simulink model "Filter_PQ_Data"  (R2018a)
settings: Solver=ode45  StartTime=0.0  StopTime=5  RelTol=1e-3  EnableMultiTasking=on
Description:
  | Copyright 2014-2018 The MathWorks, Inc.
settings Model: Creator=smiller  LastModifiedBy=smiller
settings DataIOCC: LimitDataPoints=on  SaveFormat=Array
settings OptimizationCC: LifeSpan=inf
settings DebuggingCC: UnderspecifiedInitializationDetection=Classic  MergeDetectMultiDrivingBlocksExec=none  SolverPrmCheckMsg=warning  AllowSymbolicDim=off  StateNameClashWarn=warning  SFUnexpectedBacktrackingDiag=warning  SFNoUnconditionalDefaultTransitionDiag=warning  SFExecutionAtInitializationDiag=none
settings HardwareCC: ProdBitPerPointer=32  ProdBitPerSizeT=32  ProdBitPerPtrDiffT=32  ProdLargestAtomicFloat=None  ProdIntDivRoundTo=Undefined  ProdEndianess=Unspecified  ProdWordSize=32  ProdHWDeviceType=32-bit Generic
settings ModelReferenceCC: PropagateSignalLabelsOutOfModel=off
settings CodeAppCC: StateflowObjectComments=on
settings GRTTargetCC: TargetLangStandard=C89/C90 (ANSI)  GeneratePreprocessorConditionals=Disable all
settings ConfigComp: CovMetricSettings=dw  CovHtmlReporting=on  CovSaveCumulativeToWorkspaceVar=on  CovSaveSingleToWorkspaceVar=on  CovExternalEMLEnable=off  CovSFcnEnable=off

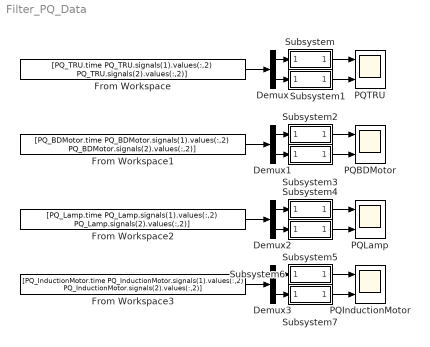
== system Filter_PQ_Data ==
  Demux{,1..3} (4 alike) : Demux  Outputs=2
  From Workspace : FromWorkspace  VariableName=[PQ_TRU.time PQ_TRU.signals(1).values(:,2) PQ_TRU.signals(2).values(:,2)]  SampleTime=0
  From Workspace1 : FromWorkspace  VariableName=[PQ_BDMotor.time PQ_BDMotor.signals(1).values(:,2) PQ_BDMotor.signals(2).values(:,2)]  SampleTime=0
  From Workspace2 : FromWorkspace  VariableName=[PQ_Lamp.time PQ_Lamp.signals(1).values(:,2) PQ_Lamp.signals(2).values(:,2)]  SampleTime=0
  From Workspace3 : FromWorkspace  VariableName=[PQ_InductionMotor.time PQ_InductionMotor.signals(1).values(:,2) PQ_InductionMotor.signals(2).values(:,2)]  SampleTime=0
  PQBDMotor : Scope  NumInputPorts=2
  PQInductionMotor : Scope  NumInputPorts=2
  PQLamp : Scope  NumInputPorts=2
  PQTRU : Scope  NumInputPorts=2
  Subsystem : Subsystem
  Subsystem1 : Subsystem
  Subsystem2 : Subsystem
  Subsystem3 : Subsystem
  Subsystem4 : Subsystem
  Subsystem5 : Subsystem
  Subsystem6 : Subsystem
  Subsystem7 : Subsystem
  wires:
  Subsystem/1(Out1) -> PQTRU/1
  Subsystem1/1(Out1) -> PQTRU/2
  Subsystem2/1(Out1) -> PQBDMotor/1
  Subsystem3/1(Out1) -> PQBDMotor/2
  From Workspace/1 -> Demux/1
  Demux/1 -> Subsystem/1(In1)
  Demux/2 -> Subsystem1/1(In1)
  From Workspace1/1 -> Demux1/1
  Demux1/1 -> Subsystem2/1(In1)
  Demux1/2 -> Subsystem3/1(In1)
  Subsystem4/1(Out1) -> PQLamp/1
  Subsystem5/1(Out1) -> PQLamp/2
  From Workspace2/1 -> Demux2/1
  Demux2/1 -> Subsystem4/1(In1)
  Demux2/2 -> Subsystem5/1(In1)
  Subsystem6/1(Out1) -> PQInductionMotor/1
  Subsystem7/1(Out1) -> PQInductionMotor/2
  From Workspace3/1 -> Demux3/1
  Demux3/1 -> Subsystem6/1(In1)
  Demux3/2 -> Subsystem7/1(In1)

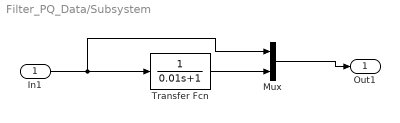
== system Filter_PQ_Data/Subsystem ==
  In1 : Inport
  Mux : Mux  Inputs=2
  Transfer Fcn : TransferFcn  Denominator=[0.01 1]
  Out1 : Outport
  wires:
  Mux/1 -> Out1/1
  In1/1 -> Mux/1, Transfer Fcn/1
  Transfer Fcn/1 -> Mux/2

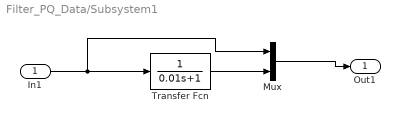
== system Filter_PQ_Data/Subsystem1 ==
  In1 : Inport
  Mux : Mux  Inputs=2
  Transfer Fcn : TransferFcn  Denominator=[0.01 1]
  Out1 : Outport
  wires:
  Transfer Fcn/1 -> Mux/2
  In1/1 -> Transfer Fcn/1, Mux/1
  Mux/1 -> Out1/1

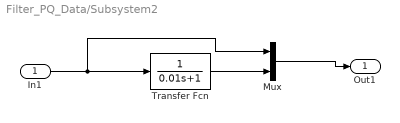
== system Filter_PQ_Data/Subsystem2 ==
  In1 : Inport
  Mux : Mux  Inputs=2
  Transfer Fcn : TransferFcn  Denominator=[0.01 1]
  Out1 : Outport
  wires:
  Transfer Fcn/1 -> Mux/2
  In1/1 -> Transfer Fcn/1, Mux/1
  Mux/1 -> Out1/1

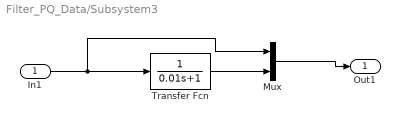
== system Filter_PQ_Data/Subsystem3 ==
  In1 : Inport
  Mux : Mux  Inputs=2
  Transfer Fcn : TransferFcn  Denominator=[0.01 1]
  Out1 : Outport
  wires:
  Mux/1 -> Out1/1
  In1/1 -> Mux/1, Transfer Fcn/1
  Transfer Fcn/1 -> Mux/2

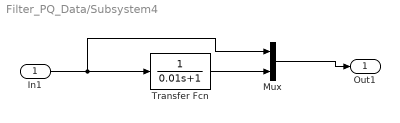
== system Filter_PQ_Data/Subsystem4 ==
  In1 : Inport
  Mux : Mux  Inputs=2
  Transfer Fcn : TransferFcn  Denominator=[0.01 1]
  Out1 : Outport
  wires:
  Mux/1 -> Out1/1
  In1/1 -> Mux/1, Transfer Fcn/1
  Transfer Fcn/1 -> Mux/2

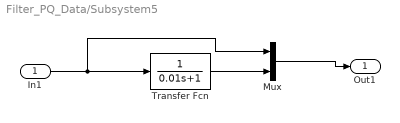
== system Filter_PQ_Data/Subsystem5 ==
  In1 : Inport
  Mux : Mux  Inputs=2
  Transfer Fcn : TransferFcn  Denominator=[0.01 1]
  Out1 : Outport
  wires:
  Transfer Fcn/1 -> Mux/2
  In1/1 -> Transfer Fcn/1, Mux/1
  Mux/1 -> Out1/1

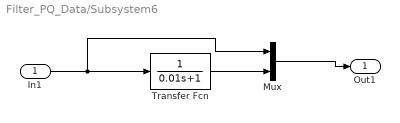
== system Filter_PQ_Data/Subsystem6 ==
  In1 : Inport
  Mux : Mux  Inputs=2
  Transfer Fcn : TransferFcn  Denominator=[0.01 1]
  Out1 : Outport
  wires:
  Transfer Fcn/1 -> Mux/2
  In1/1 -> Transfer Fcn/1, Mux/1
  Mux/1 -> Out1/1

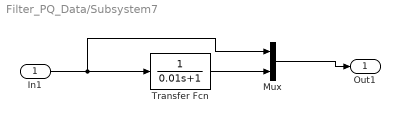
== system Filter_PQ_Data/Subsystem7 ==
  In1 : Inport
  Mux : Mux  Inputs=2
  Transfer Fcn : TransferFcn  Denominator=[0.01 1]
  Out1 : Outport
  wires:
  Mux/1 -> Out1/1
  In1/1 -> Mux/1, Transfer Fcn/1
  Transfer Fcn/1 -> Mux/2
